simulink model "clik_transp"  (R2023b)
settings: Solver=VariableStepAuto  StartTime=0.0  StopTime=50  RelTol=1e-3
undefined symbols (not defined in the file or in its folder): DiscIntNeverNeededParam, K_trasp, q0, Tc
settings Model: Creator=fiore  LastModifiedBy=fiore

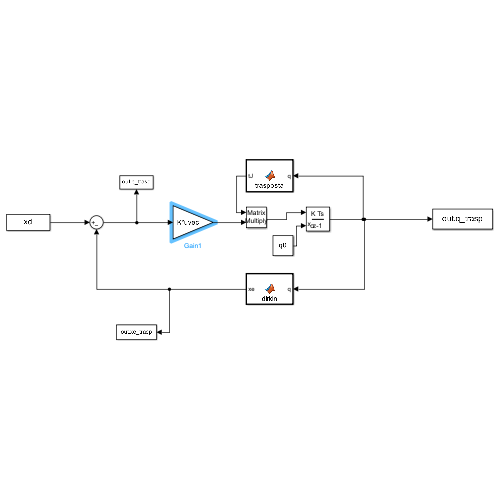
[thumbnail: Simulink's stored preview of the top-level diagram]
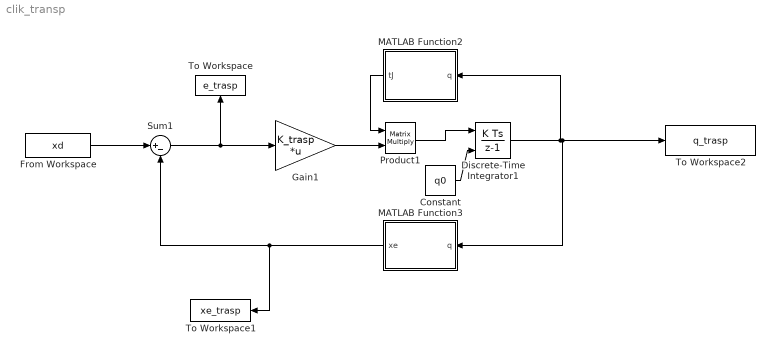
== system clik_transp ==
  Constant : Constant  Value=q0
  Discrete-Time Integrator1 : DiscreteIntegrator  InitialConditionSource=external  InitialCondition=q0  SampleTime=Tc  ICPrevOutput=DiscIntNeverNeededParam  ICPrevScaledInput=DiscIntNeverNeededParam
  From Workspace : FromWorkspace  VariableName=xd  SampleTime=Tc
  Gain1 : Gain  Gain=K_trasp  Multiplication=Matrix(K*u) (u vector)
  MATLAB Function2 : MATLAB Function  TreatAsAtomicUnit=on
  MATLAB Function3 : MATLAB Function  TreatAsAtomicUnit=on
  Product1 : Product  Multiplication=Matrix(*)
  Sum1 : Sum  Inputs=|+-
  To Workspace : ToWorkspace  VariableName=e_trasp  SaveFormat=Structure With Time  SampleTime=-1
  To Workspace1 : ToWorkspace  VariableName=xe_trasp  SaveFormat=Structure With Time  SampleTime=-1
  To Workspace2 : ToWorkspace  VariableName=q_trasp  SaveFormat=Structure With Time  SampleTime=-1
  wires:
  MATLAB Function3/1(xe) -> Sum1/2, To Workspace1/1
  Sum1/1 -> To Workspace/1, Gain1/1
  MATLAB Function2/1(tJ) -> Product1/1
  Discrete-Time Integrator1/1 -> MATLAB Function3/1(q), To Workspace2/1, MATLAB Function2/1(q)
  Gain1/1 -> Product1/2
  Product1/1 -> Discrete-Time Integrator1/1
  From Workspace/1 -> Sum1/1
  Constant/1 -> Discrete-Time Integrator1/2

== matlab function clik_transp/MATLAB Function3 ==
  data: q input; xe output
function xe = dirkin(q)
a1=0.5;
a2=a1;
d0=1;


xe=[a1*cos(q(1))+a2*cos(q(1)+q(2));...
    a1*sin(q(1))+a2*sin(q(1)+q(2));...
    d0+q(3);...
    q(1)+q(2)+q(4)];
end

== matlab function clik_transp/MATLAB Function2 ==
  data: tJ output; q input
function tJ=trasposta(q)
a1=0.5;
a2=a1;

J=[-a1*sin(q(1))-a2*sin(q(1)+q(2)),-a2*sin(q(1)+q(2)),0,0;...
    a1*cos(q(1))+a2*cos(q(1)+q(2)),a2*cos(q(1)+q(2)),0,0;...
    0,0,1,0;...
    1,1,0,1];
tJ=J';
end
